simulink model "BasicMotorModelTest"  (R2020b)
settings: Solver=VariableStepAuto  StartTime=0.0  StopTime=20  RelTol=1e-3
libraries: simulink x1
settings Model: Creator=janse  LastModifiedBy=janse

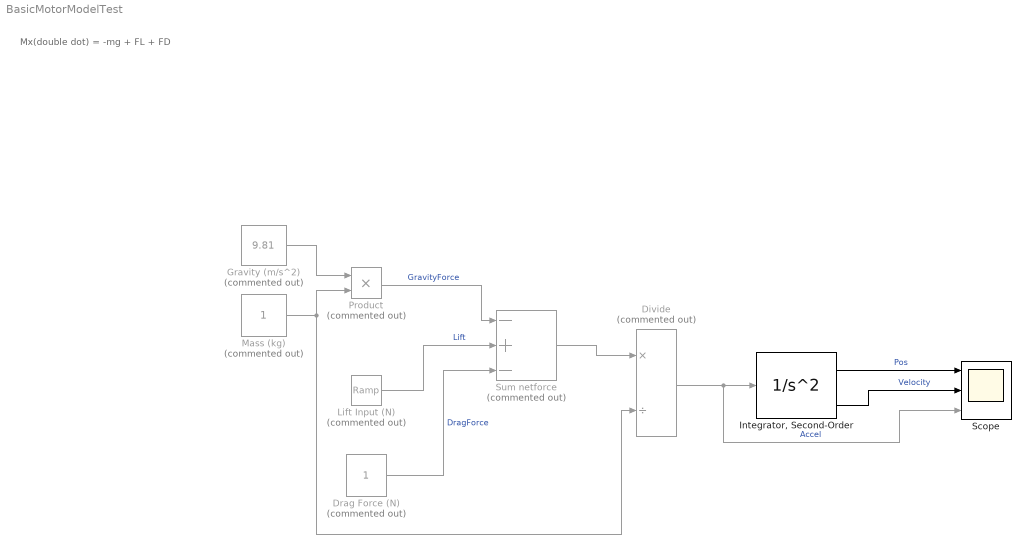
== system BasicMotorModelTest ==
  note: Mx(double dot) = -mg + FL + FD
  Divide : Product  Commented=on  Inputs=*/
  Drag Force (N) : Constant  Commented=on
  Gravity (m/s^2) : Constant  Commented=on  Value=9.81
  "Integrator, Second-Order" : SecondOrderIntegrator
  Lift Input (N) : simulink/Sources/Ramp  Commented=on  slope=2  start=0  InitialOutput=0
  Mass (kg) : Constant  Commented=on
  Product : Product  Commented=on
  Scope : Scope  NumInputPorts=3
  "Sum netforce " : Sum  Commented=on  Inputs=-+-
  wires:
  Gravity (m/s^2)/1 -> Product/1
  Product/1 -> "Sum netforce "/1  "GravityForce"
  Lift Input (N)/1 -> "Sum netforce "/2  "Lift"
  Drag Force (N)/1 -> "Sum netforce "/3  "DragForce"
  "Sum netforce "/1 -> Divide/1
  Mass (kg)/1 -> Divide/2, Product/2
  Divide/1 -> "Integrator, Second-Order"/1, Scope/3  "Accel"
  "Integrator, Second-Order"/1 -> Scope/1  "Pos"
  "Integrator, Second-Order"/2 -> Scope/2  "Velocity"
